simulink model "SF054A_PwrpkCmpbltyChk"  (R2013b)
settings: Solver=FixedStepDiscrete  SolverMode=SingleTasking  StartTime=0.0  StopTime=1  FixedStep=0.1  RelTol=1e-3
values from neighbouring files (symbols this model uses):
  CNVTOCNT_CNTPERMILLISEC_U32 = DataDict.Constant    [SF054A_PwrpkCmpbltyChk_DataDict.m]
  CORRLNFLTBIT2_CNT_U08 = DataDict.Constant    [SF054A_PwrpkCmpbltyChk_DataDict.m]
  CORRLNGEARIDFLTBIT3_CNT_U08 = DataDict.Constant    [SF054A_PwrpkCmpbltyChk_DataDict.m]
  GEARID1INVLBIT0_CNT_U08 = DataDict.Constant    [SF054A_PwrpkCmpbltyChk_DataDict.m]
  GEARID2INVLBIT1_CNT_U08 = DataDict.Constant    [SF054A_PwrpkCmpbltyChk_DataDict.m]
  NODEBSTEP_CNT_U16 = DataDict.Constant    [SF054A_PwrpkCmpbltyChk_DataDict.m]
  NOFAULT_CNT_U08 = DataDict.Constant    [SF054A_PwrpkCmpbltyChk_DataDict.m]
  PwrpkCmpbltyChkGearId = DataDict.Calibration    [SF054A_PwrpkCmpbltyChk_DataDict.m]
  TMRTHD_MILLISEC_U32 = DataDict.Constant    [SF054A_PwrpkCmpbltyChk_DataDict.m]
undefined symbols (not defined in the file or in its folder): NtcNr1, NtcSts1, SigQlfr1
libraries: simulink x10
(part 2 of 3)

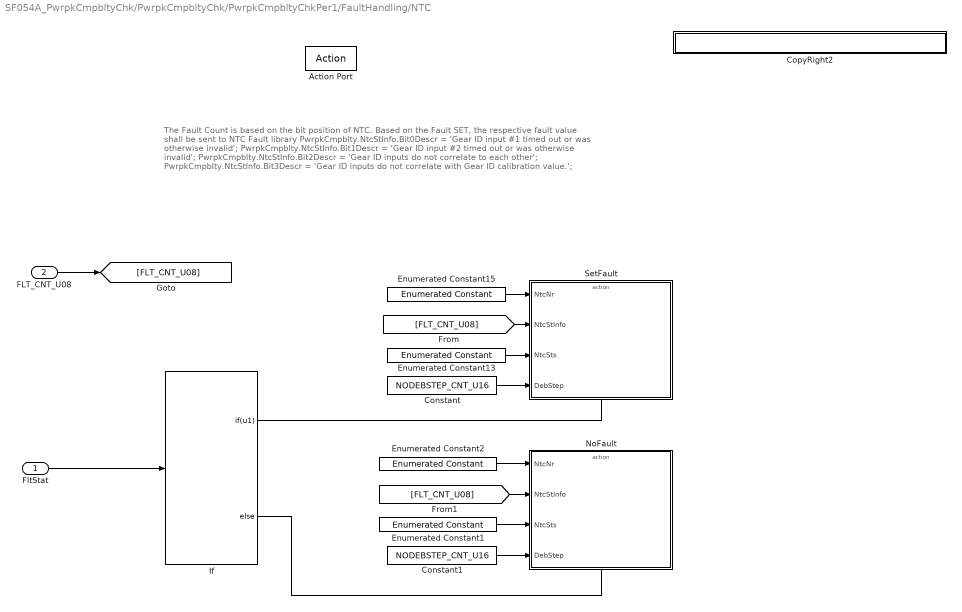
== system SF054A_PwrpkCmpbltyChk/PwrpkCmpbltyChk/PwrpkCmpbltyChkPer1/FaultHandling/NTC ==
  note: The Fault Count is based on the bit position of NTC. Based on the Fault SET, the respective fault value shall be sent to NTC Fault library
      |
      | PwrpkCmpblty.NtcStInfo.Bit0Descr = 'Gear ID input #1 timed out or was otherwise invalid';
      | PwrpkCmpblty.NtcStInfo.Bit1Descr = 'Gear ID input #2 timed out or was otherwise invalid';
      | PwrpkCmpblty.NtcStInfo.Bit2Descr = 'Gear ID inputs do not correlate to each other';
      | PwrpkCmpblty.NtcStInfo.Bit3Descr = 'Gear ID inputs do not correlate with Gear ID calibration value.';
  FltStat : Inport  RequirementInfo="{'linktype_rmi_doors' '0000baba (/E-STEER Core/SubSystem Specifications/Application Functions/SF054A Powerpack Compatibility Check)' '#SF054A_94' 'true' 'REQ:  SF054A_94' '' ; 'linktype_rmi_doors' '0000baba (/E-STEER Core/SubSystem Specifications/Application Functions/SF054A Powerpack Compatibility Check)' '#SF054A_95' 'true' 'REQ:  SF054A_95' '' ; 'linktype_rmi_doors' '0000baba (/E-STEER Core/SubSystem Specifications/Application Functions/SF054A Powerpack Compatibility Check)' '#SF054A_96' 'true' 'REQ:  SF054A_96' '' } %GIDa_d1321426_f376_4e74_abf1_ce402bb86bea"
  FLT_CNT_U08 : Inport  RequirementInfo="{'linktype_rmi_doors' '0000baba (/E-STEER Core/SubSystem Specifications/Application Functions/SF054A Powerpack Compatibility Check)' '#SF054A_94' 'true' 'REQ:  SF054A_94' '' ; 'linktype_rmi_doors' '0000baba (/E-STEER Core/SubSystem Specifications/Application Functions/SF054A Powerpack Compatibility Check)' '#SF054A_95' 'true' 'REQ:  SF054A_95' '' ; 'linktype_rmi_doors' '0000baba (/E-STEER Core/SubSystem Specifications/Application Functions/SF054A Powerpack Compatibility Check)' '#SF054A_96' 'true' 'REQ:  SF054A_96' '' } %GIDa_a4ede8dd_1dc7_48ae_adab_c593f70f9e10"  Port=2
  Action Port : ActionPort  ActionType=then
  Constant : Constant  Value=NODEBSTEP_CNT_U16
  Constant1 : Constant  Value=NODEBSTEP_CNT_U16
  CopyRight2 : Subsystem  Description=|  mask(Copyright Information){none=on}
      | Copyright info block.                                               
      |                                                                     
      | Place copyright information at the top of every subsystem in design.
      mask prompts: none "No parameters"
      mask help: Place copyright information at the top of every subsystem in design.
      mask Display:
      | NxtrConf = 'Nexteer Confidential';
      | 
      | sys = bdroot; %handle for the current model ("system")
      | first = get_param(sys,'Created');
      | if(isempty(first))
      |     first = datestr(now,'yyyy');
      | else
      |     first = first(end-3:end);  %year is last four digits
      | end
      | 
      | last = get_param(sys,'LastModifiedDate');
      | if isempty(last)
      |     last = datestr(now,'yyyy');
      | else
      |     last = last(end-3:end);
      | end
      | 
      | if strcmp(first,last)
      |     fprintf('%s -- Copyright %s Nexteer',NxtrConf,first)
      | else
      |     fprintf('%s -- %s%s- %s Nexteer',NxtrConf,char(169),first,last)
      | end
  Enumerated Constant1 : simulink/Sources/Enumerated Constant  RequirementInfo="{'linktype_rmi_doors' '0000ba59 (/E-STEER Core/SubSystem Specifications/Application Functions/SF011A Learned EOT Limits)' '#SF011A_147' 'true' 'REQ:  SF011A_147' '' ; 'linktype_rmi_doors' '0000baba (/E-STEER Core/SubSystem Specifications/Application Functions/SF054A Powerpack Compatibility Check)' '#SF054A_94' 'true' 'REQ:  SF054A_94' '' ; 'linktype_rmi_doors' '0000baba (/E-STEER Core/SubSystem Specifications/Application Functions/SF054A Powerpack Compatibility Check)' '#SF054A_95' 'true' 'REQ:  SF054A_95' '' ; 'linktype_rmi_doors' '0000baba (/E-STEER Core/SubSystem Specifications/Application Functions/SF054A Powerpack Compatibility Check)' '#SF054A_96' 'true' 'REQ:  SF054A_96' '' ; 'linktype_rmi_doors' '0000baba (/E-STEER Core/SubSystem Specifications/Application Functions/SF054A Powerpack Compatibility Check)' '#SF054A_93' 'true' 'REQ:  SF054A_93' '' ; 'linktype_rmi_doors' '0000baba (/E-STEER Core/SubSystem Specifications/Application Functions/SF054A Powerpack Compatibility Check)' '#SF054A_97' 'true' 'REQ:  SF054A_97' '' } %GIDa_76a10143_d7e5_4556_a877_13f786568e17"  OutDataTypeStr=Enum: NtcSts1  Value=NtcSts1.NTCSTS_PASSD  SampleTime=inf
  Enumerated Constant13 : simulink/Sources/Enumerated Constant  RequirementInfo="{'linktype_rmi_doors' '0000ba59 (/E-STEER Core/SubSystem Specifications/Application Functions/SF011A Learned EOT Limits)' '#SF011A_147' 'true' 'REQ:  SF011A_147' '' ; 'linktype_rmi_doors' '0000baba (/E-STEER Core/SubSystem Specifications/Application Functions/SF054A Powerpack Compatibility Check)' '#SF054A_94' 'true' 'REQ:  SF054A_94' '' ; 'linktype_rmi_doors' '0000baba (/E-STEER Core/SubSystem Specifications/Application Functions/SF054A Powerpack Compatibility Check)' '#SF054A_95' 'true' 'REQ:  SF054A_95' '' ; 'linktype_rmi_doors' '0000baba (/E-STEER Core/SubSystem Specifications/Application Functions/SF054A Powerpack Compatibility Check)' '#SF054A_96' 'true' 'REQ:  SF054A_96' '' } %GIDa_90bc376e_b768_4a6f_b02b_6410e016d981"  OutDataTypeStr=Enum: NtcSts1  Value=NtcSts1.NTCSTS_FAILD  SampleTime=inf
  Enumerated Constant15 : simulink/Sources/Enumerated Constant  RequirementInfo="{'linktype_rmi_doors' '0000ba59 (/E-STEER Core/SubSystem Specifications/Application Functions/SF011A Learned EOT Limits)' '#SF011A_147' 'true' 'REQ:  SF011A_147' '' } %GIDa_98664301_0d49_4c1a_b13b_e4ddba13ec9c"  OutDataTypeStr=Enum: NtcNr1  Value=NtcNr1.NTCNR_0X1F1  SampleTime=inf
  Enumerated Constant2 : simulink/Sources/Enumerated Constant  RequirementInfo="{'linktype_rmi_doors' '0000ba59 (/E-STEER Core/SubSystem Specifications/Application Functions/SF011A Learned EOT Limits)' '#SF011A_147' 'true' 'REQ:  SF011A_147' '' ; 'linktype_rmi_doors' '0000baba (/E-STEER Core/SubSystem Specifications/Application Functions/SF054A Powerpack Compatibility Check)' '#SF054A_94' 'true' 'REQ:  SF054A_94' '' ; 'linktype_rmi_doors' '0000baba (/E-STEER Core/SubSystem Specifications/Application Functions/SF054A Powerpack Compatibility Check)' '#SF054A_95' 'true' 'REQ:  SF054A_95' '' ; 'linktype_rmi_doors' '0000baba (/E-STEER Core/SubSystem Specifications/Application Functions/SF054A Powerpack Compatibility Check)' '#SF054A_96' 'true' 'REQ:  SF054A_96' '' ; 'linktype_rmi_doors' '0000baba (/E-STEER Core/SubSystem Specifications/Application Functions/SF054A Powerpack Compatibility Check)' '#SF054A_93' 'true' 'REQ:  SF054A_93' '' ; 'linktype_rmi_doors' '0000baba (/E-STEER Core/SubSystem Specifications/Application Functions/SF054A Powerpack Compatibility Check)' '#SF054A_97' 'true' 'REQ:  SF054A_97' '' } %GIDa_e47249a4_767f_41c6_83fc_25906c6d5740"  OutDataTypeStr=Enum: NtcNr1  Value=NtcNr1.NTCNR_0X1F1  SampleTime=inf
  If : If  RequirementInfo="{'linktype_rmi_doors' '0000baba (/E-STEER Core/SubSystem Specifications/Application Functions/SF054A Powerpack Compatibility Check)' '#SF054A_93' 'true' 'REQ:  SF054A_93' '' ; 'linktype_rmi_doors' '0000baba (/E-STEER Core/SubSystem Specifications/Application Functions/SF054A Powerpack Compatibility Check)' '#SF054A_97' 'true' 'REQ:  SF054A_97' '' ; 'linktype_rmi_doors' '0000baba (/E-STEER Core/SubSystem Specifications/Application Functions/SF054A Powerpack Compatibility Check)' '#SF054A_94' 'true' 'REQ:  SF054A_94' '' ; 'linktype_rmi_doors' '0000baba (/E-STEER Core/SubSystem Specifications/Application Functions/SF054A Powerpack Compatibility Check)' '#SF054A_95' 'true' 'REQ:  SF054A_95' '' ; 'linktype_rmi_doors' '0000baba (/E-STEER Core/SubSystem Specifications/Application Functions/SF054A Powerpack Compatibility Check)' '#SF054A_96' 'true' 'REQ:  SF054A_96' '' } %GIDa_5ebd1fa8_c02e_40bb_a2aa_3fc1e27259c9"  IfExpression=u1
  NoFault : Subsystem  RequirementInfo="{'linktype_rmi_doors' '0000baba (/E-STEER Core/SubSystem Specifications/Application Functions/SF054A Powerpack Compatibility Check)' '#SF054A_94' 'true' 'REQ:  SF054A_94' '' ; 'linktype_rmi_doors' '0000baba (/E-STEER Core/SubSystem Specifications/Application Functions/SF054A Powerpack Compatibility Check)' '#SF054A_95' 'true' 'REQ:  SF054A_95' '' ; 'linktype_rmi_doors' '0000baba (/E-STEER Core/SubSystem Specifications/Application Functions/SF054A Powerpack Compatibility Check)' '#SF054A_96' 'true' 'REQ:  SF054A_96' '' ; 'linktype_rmi_doors' '0000baba (/E-STEER Core/SubSystem Specifications/Application Functions/SF054A Powerpack Compatibility Check)' '#SF054A_93' 'true' 'REQ:  SF054A_93' '' ; 'linktype_rmi_doors' '0000baba (/E-STEER Core/SubSystem Specifications/Application Functions/SF054A Powerpack Compatibility Check)' '#SF054A_97' 'true' 'REQ:  SF054A_97' '' } %GIDa_9ffc1e70_19a3_4cc1_b8dc_1508988df6dd"  mask(SetNTC){}
      mask help: SetNTC library block
  SetFault : Subsystem  RequirementInfo="{'linktype_rmi_doors' '0000baba (/E-STEER Core/SubSystem Specifications/Application Functions/SF054A Powerpack Compatibility Check)' '#SF054A_93' 'true' 'REQ:  SF054A_93' '' ; 'linktype_rmi_doors' '0000baba (/E-STEER Core/SubSystem Specifications/Application Functions/SF054A Powerpack Compatibility Check)' '#SF054A_97' 'true' 'REQ:  SF054A_97' '' ; 'linktype_rmi_doors' '0000baba (/E-STEER Core/SubSystem Specifications/Application Functions/SF054A Powerpack Compatibility Check)' '#SF054A_94' 'true' 'REQ:  SF054A_94' '' ; 'linktype_rmi_doors' '0000baba (/E-STEER Core/SubSystem Specifications/Application Functions/SF054A Powerpack Compatibility Check)' '#SF054A_95' 'true' 'REQ:  SF054A_95' '' ; 'linktype_rmi_doors' '0000baba (/E-STEER Core/SubSystem Specifications/Application Functions/SF054A Powerpack Compatibility Check)' '#SF054A_96' 'true' 'REQ:  SF054A_96' '' } %GIDa_5c8bf209_0d3d_49fa_8c93_879ef1e5ed4e"  mask(SetNTC){}
      mask help: SetNTC library block
  wires:
  Enumerated Constant15/1 -> SetFault/1(NtcNr)
  Enumerated Constant13/1 -> SetFault/3(NtcSts)
  Constant/1 -> SetFault/4(DebStep)
  [FLT_CNT_U08] -> SetFault/2(NtcStInfo)
  If/1 -> SetFault/Action
  Enumerated Constant2/1 -> NoFault/1(NtcNr)
  Enumerated Constant1/1 -> NoFault/3(NtcSts)
  Constant1/1 -> NoFault/4(DebStep)
  [FLT_CNT_U08] -> NoFault/2(NtcStInfo)
  If/2 -> NoFault/Action
  FltStat/1 -> If/1
  FLT_CNT_U08/1 -> [FLT_CNT_U08]

== system SF054A_PwrpkCmpbltyChk/PwrpkCmpbltyChk/PwrpkCmpbltyChkPer1/FaultHandling/NTCCheck ==
  FltStat : Inport  RequirementInfo="{'linktype_rmi_doors' '0000baba (/E-STEER Core/SubSystem Specifications/Application Functions/SF054A Powerpack Compatibility Check)' '#SF054A_91' 'true' 'REQ:  SF054A_91' '' ; 'linktype_rmi_doors' '0000baba (/E-STEER Core/SubSystem Specifications/Application Functions/SF054A Powerpack Compatibility Check)' '#SF054A_98' 'true' 'REQ:  SF054A_98' '' } %GIDa_cd991dcd_1012_4078_b2f9_adfb3d5191aa"
  Constant : Constant  RequirementInfo="{'linktype_rmi_doors' '0000baba (/E-STEER Core/SubSystem Specifications/Application Functions/SF054A Powerpack Compatibility Check)' '#SF054A_91' 'true' 'REQ:  SF054A_91' '' ; 'linktype_rmi_doors' '0000baba (/E-STEER Core/SubSystem Specifications/Application Functions/SF054A Powerpack Compatibility Check)' '#SF054A_98' 'true' 'REQ:  SF054A_98' '' } %GIDa_b6b6c8fe_27bd_4710_8193_37bbd19d7a9e"
  Enumerated Constant1 : simulink/Sources/Enumerated Constant  RequirementInfo="{'linktype_rmi_doors' '0000baba (/E-STEER Core/SubSystem Specifications/Application Functions/SF054A Powerpack Compatibility Check)' '#SF054A_91' 'true' 'REQ:  SF054A_91' '' ; 'linktype_rmi_doors' '0000baba (/E-STEER Core/SubSystem Specifications/Application Functions/SF054A Powerpack Compatibility Check)' '#SF054A_98' 'true' 'REQ:  SF054A_98' '' } %GIDa_7ed6285f_7121_49e3_927a_e109339fc9b9"  OutDataTypeStr=Enum: SigQlfr1  Value=SigQlfr1.SIGQLFR_PASSD  SampleTime=inf
  Enumerated Constant3 : simulink/Sources/Enumerated Constant  RequirementInfo="{'linktype_rmi_doors' '0000baba (/E-STEER Core/SubSystem Specifications/Application Functions/SF054A Powerpack Compatibility Check)' '#SF054A_91' 'true' 'REQ:  SF054A_91' '' ; 'linktype_rmi_doors' '0000baba (/E-STEER Core/SubSystem Specifications/Application Functions/SF054A Powerpack Compatibility Check)' '#SF054A_98' 'true' 'REQ:  SF054A_98' '' } %GIDa_ae37c846_cbb7_4a30_8716_1da98cb1c54b"  OutDataTypeStr=Enum: NtcNr1  Value=NtcNr1.NTCNR_0X1F1  SampleTime=inf
  Enumerated Constant4 : simulink/Sources/Enumerated Constant  RequirementInfo="{'linktype_rmi_doors' '0000baba (/E-STEER Core/SubSystem Specifications/Application Functions/SF054A Powerpack Compatibility Check)' '#SF054A_91' 'true' 'REQ:  SF054A_91' '' ; 'linktype_rmi_doors' '0000baba (/E-STEER Core/SubSystem Specifications/Application Functions/SF054A Powerpack Compatibility Check)' '#SF054A_98' 'true' 'REQ:  SF054A_98' '' } %GIDa_9ccbda32_b0ec_468a_9ed5_5f897a56dcc4"  OutDataTypeStr=Enum: SigQlfr1  Value=SigQlfr1.SIGQLFR_PASSD  SampleTime=inf
  GetNtcQlfrSts : Subsystem  RequirementInfo="{'linktype_rmi_doors' '0000baba (/E-STEER Core/SubSystem Specifications/Application Functions/SF054A Powerpack Compatibility Check)' '#SF054A_91' 'true' 'REQ:  SF054A_91' '' ; 'linktype_rmi_doors' '0000baba (/E-STEER Core/SubSystem Specifications/Application Functions/SF054A Powerpack Compatibility Check)' '#SF054A_98' 'true' 'REQ:  SF054A_98' '' } %GIDa_63a61b2e_15bc_4085_be85_8a45fba3da91"  Priority=0  TreatAsAtomicUnit=on  mask(GetNTC){}
      mask help: GetNTC library block
      settings: RTWSystemCode=Inline
  If : If  RequirementInfo="{'linktype_rmi_doors' '0000baba (/E-STEER Core/SubSystem Specifications/Application Functions/SF054A Powerpack Compatibility Check)' '#SF054A_91' 'true' 'REQ:  SF054A_91' '' ; 'linktype_rmi_doors' '0000baba (/E-STEER Core/SubSystem Specifications/Application Functions/SF054A Powerpack Compatibility Check)' '#SF054A_98' 'true' 'REQ:  SF054A_98' '' } %GIDa_6f272258_94a1_4eea_8ab6_e33777d6ad2e"  Priority=1  IfExpression=u1  ShowElse=off
  Logical Operator : Logic  RequirementInfo="{'linktype_rmi_doors' '0000baba (/E-STEER Core/SubSystem Specifications/Application Functions/SF054A Powerpack Compatibility Check)' '#SF054A_91' 'true' 'REQ:  SF054A_91' '' ; 'linktype_rmi_doors' '0000baba (/E-STEER Core/SubSystem Specifications/Application Functions/SF054A Powerpack Compatibility Check)' '#SF054A_98' 'true' 'REQ:  SF054A_98' '' } %GIDa_29bb41fa_cbd1_428c_8cf2_147e2dfe02ab"  Operator=OR  AllPortsSameDT=off  OutDataTypeStr=boolean
  Logical Operator1 : Logic  RequirementInfo="{'linktype_rmi_doors' '0000baba (/E-STEER Core/SubSystem Specifications/Application Functions/SF054A Powerpack Compatibility Check)' '#SF054A_91' 'true' 'REQ:  SF054A_91' '' ; 'linktype_rmi_doors' '0000baba (/E-STEER Core/SubSystem Specifications/Application Functions/SF054A Powerpack Compatibility Check)' '#SF054A_98' 'true' 'REQ:  SF054A_98' '' } %GIDa_27601766_4d47_46cd_835d_6e2f4316db1e"  AllPortsSameDT=off  OutDataTypeStr=boolean
  NtcStsChk : RelationalOperator  RequirementInfo="{'linktype_rmi_doors' '0000baba (/E-STEER Core/SubSystem Specifications/Application Functions/SF054A Powerpack Compatibility Check)' '#SF054A_91' 'true' 'REQ:  SF054A_91' '' ; 'linktype_rmi_doors' '0000baba (/E-STEER Core/SubSystem Specifications/Application Functions/SF054A Powerpack Compatibility Check)' '#SF054A_98' 'true' 'REQ:  SF054A_98' '' } %GIDa_b3194a09_2e5a_47be_940a_7a93a9f9800c"  Operator=~=  OutDataTypeStr=boolean
  NtcStsChk1 : RelationalOperator  RequirementInfo="{'linktype_rmi_doors' '0000baba (/E-STEER Core/SubSystem Specifications/Application Functions/SF054A Powerpack Compatibility Check)' '#SF054A_91' 'true' 'REQ:  SF054A_91' '' ; 'linktype_rmi_doors' '0000baba (/E-STEER Core/SubSystem Specifications/Application Functions/SF054A Powerpack Compatibility Check)' '#SF054A_98' 'true' 'REQ:  SF054A_98' '' } %GIDa_82d14e30_4785_436e_ab50_a0d52d13e43f"  Operator===  OutDataTypeStr=boolean
  NtcStsChk2 : RelationalOperator  RequirementInfo="{'linktype_rmi_doors' '0000baba (/E-STEER Core/SubSystem Specifications/Application Functions/SF054A Powerpack Compatibility Check)' '#SF054A_91' 'true' 'REQ:  SF054A_91' '' ; 'linktype_rmi_doors' '0000baba (/E-STEER Core/SubSystem Specifications/Application Functions/SF054A Powerpack Compatibility Check)' '#SF054A_98' 'true' 'REQ:  SF054A_98' '' } %GIDa_f955f7c9_8f8a_47c5_a799_e283ca9a9948"  Operator===  OutDataTypeStr=boolean
  NTC_Condition : Outport  RequirementInfo="{'linktype_rmi_doors' '0000baba (/E-STEER Core/SubSystem Specifications/Application Functions/SF054A Powerpack Compatibility Check)' '#SF054A_91' 'true' 'REQ:  SF054A_91' '' ; 'linktype_rmi_doors' '0000baba (/E-STEER Core/SubSystem Specifications/Application Functions/SF054A Powerpack Compatibility Check)' '#SF054A_98' 'true' 'REQ:  SF054A_98' '' } %GIDa_f2a5627a_783c_4d45_b613_59ba6ee0c185"
  wires:
  Enumerated Constant4/1 -> NtcStsChk/2
  Enumerated Constant3/1 -> GetNtcQlfrSts/1(NtcNr)
  GetNtcQlfrSts/1(NtcQlfr) -> NtcStsChk/1, NtcStsChk1/1
  Enumerated Constant1/1 -> NtcStsChk1/2
  NtcStsChk/1 -> Logical Operator/1
  Logical Operator/1 -> If/1
  If/1 -> NTC_Condition/1
  FltStat/1 -> NtcStsChk2/2
  Constant/1 -> NtcStsChk2/1
  NtcStsChk1/1 -> Logical Operator1/1
  NtcStsChk2/1 -> Logical Operator1/2
  Logical Operator1/1 -> Logical Operator/2

== system SF054A_PwrpkCmpbltyChk/PwrpkCmpbltyChk/PwrpkCmpbltyChkPer1/FaultDetection/CorrlnChk/CopyRight2 ==

== system SF054A_PwrpkCmpbltyChk/PwrpkCmpbltyChk/PwrpkCmpbltyChkPer1/FaultDetection/CorrlnChk/CorrlnFltChk ==
  GearIdn1 : Inport
  GearIdn2 : Inport  Port=2
  Action Port : ActionPort  ActionType=then
  CopyRight2 : Subsystem  Description=|  mask(Copyright Information){none=on}
      | Copyright info block.                                               
      |                                                                     
      | Place copyright information at the top of every subsystem in design.
      mask prompts: none "No parameters"
      mask help: Place copyright information at the top of every subsystem in design.
      mask Display:
      | NxtrConf = 'Nexteer Confidential';
      | 
      | sys = bdroot; %handle for the current model ("system")
      | first = get_param(sys,'Created');
      | if(isempty(first))
      |     first = datestr(now,'yyyy');
      | else
      |     first = first(end-3:end);  %year is last four digits
      | end
      | 
      | last = get_param(sys,'LastModifiedDate');
      | if isempty(last)
      |     last = datestr(now,'yyyy');
      | else
      |     last = last(end-3:end);
      | end
      | 
      | if strcmp(first,last)
      |     fprintf('%s -- Copyright %s Nexteer',NxtrConf,first)
      | else
      |     fprintf('%s -- %s%s- %s Nexteer',NxtrConf,char(169),first,last)
      | end
  GearIdCorrlnChk : Subsystem  RequirementInfo="{'linktype_rmi_doors' '0000baba (/E-STEER Core/SubSystem Specifications/Application Functions/SF054A Powerpack Compatibility Check)' '#SF054A_69' 'true' 'REQ:  SF054A_69' '' } %GIDa_fbed16ac_51b0_425e_93d9_51fb01c78695"  TreatAsAtomicUnit=on
  SigCorrlnChk : Subsystem  RequirementInfo="{'linktype_rmi_doors' '0000baba (/E-STEER Core/SubSystem Specifications/Application Functions/SF054A Powerpack Compatibility Check)' '#SF054A_67' 'true' 'REQ:  SF054A_67' '' } %GIDa_4edc7e58_d267_41ea_8f9b_2f7686a22c38"  TreatAsAtomicUnit=on
  GearIdCorrlnFltStat : Outport
  CorrlnFltStat : Outport  Port=2
  CorrlnFltCnt : Outport  Port=3
  GearIdCorrlnFltCnt : Outport  Port=4
  wires:
  GearIdn2/1 -> GearIdCorrlnChk/1(GearIdn2), SigCorrlnChk/2(GearIdn2)
  GearIdn1/1 -> GearIdCorrlnChk/2(GearIdn1), SigCorrlnChk/1(GearIdn1)
  GearIdCorrlnChk/1(GearIdCorrlnFltStat) -> GearIdCorrlnFltStat/1
  SigCorrlnChk/1(CorrlnFltStat) -> CorrlnFltStat/1
  SigCorrlnChk/2(CorrlnFltCnt) -> CorrlnFltCnt/1
  GearIdCorrlnChk/2(GearIdCorrlnFltCnt) -> GearIdCorrlnFltCnt/1

== system SF054A_PwrpkCmpbltyChk/PwrpkCmpbltyChk/PwrpkCmpbltyChkPer1/FaultDetection/CorrlnChk/Default ==
  Action Port : ActionPort  ActionType=else
  Constant : Constant  Value=false  OutDataTypeStr=boolean
  Constant1 : Constant  Value=false  OutDataTypeStr=boolean
  Constant2 : Constant  Value=0  OutDataTypeStr=uint8
  Constant3 : Constant  Value=0  OutDataTypeStr=uint8
  CopyRight2 : Subsystem  Description=|  mask(Copyright Information){none=on}
      | Copyright info block.                                               
      |                                                                     
      | Place copyright information at the top of every subsystem in design.
      mask prompts: none "No parameters"
      mask help: Place copyright information at the top of every subsystem in design.
      mask Display:
      | NxtrConf = 'Nexteer Confidential';
      | 
      | sys = bdroot; %handle for the current model ("system")
      | first = get_param(sys,'Created');
      | if(isempty(first))
      |     first = datestr(now,'yyyy');
      | else
      |     first = first(end-3:end);  %year is last four digits
      | end
      | 
      | last = get_param(sys,'LastModifiedDate');
      | if isempty(last)
      |     last = datestr(now,'yyyy');
      | else
      |     last = last(end-3:end);
      | end
      | 
      | if strcmp(first,last)
      |     fprintf('%s -- Copyright %s Nexteer',NxtrConf,first)
      | else
      |     fprintf('%s -- %s%s- %s Nexteer',NxtrConf,char(169),first,last)
      | end
  GearIdCorrlnFltCnt : Outport
  CorrlnFltCnt : Outport  Port=2
  CorrlnFltStat : Outport  Port=3
  GearIdCorrlnFltStat : Outport  Port=4
  wires:
  Constant/1 -> CorrlnFltStat/1
  Constant1/1 -> GearIdCorrlnFltStat/1
  Constant2/1 -> CorrlnFltCnt/1
  Constant3/1 -> GearIdCorrlnFltCnt/1

== system SF054A_PwrpkCmpbltyChk/PwrpkCmpbltyChk/PwrpkCmpbltyChkPer1/FaultDetection/GearSigChk/CopyRight2 ==

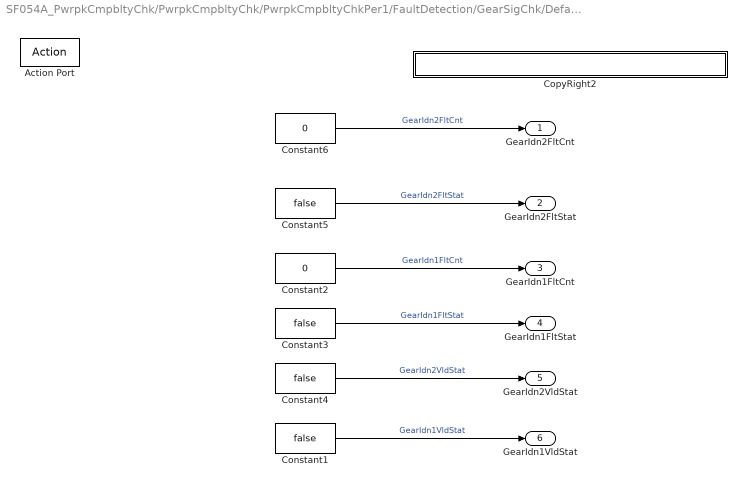
== system SF054A_PwrpkCmpbltyChk/PwrpkCmpbltyChk/PwrpkCmpbltyChkPer1/FaultDetection/GearSigChk/Default ==
  Action Port : ActionPort  ActionType=else
  Constant{1,3..5} (4 alike) : Constant  Value=false  OutDataTypeStr=boolean
      settings: AttributesFormatString=%<OutDataTypeStr>
  Constant2 : Constant  Value=0  OutDataTypeStr=uint8
      settings: AttributesFormatString=%<OutDataTypeStr>
  Constant6 : Constant  Value=0  OutDataTypeStr=uint8
      settings: AttributesFormatString=%<OutDataTypeStr>
  CopyRight2 : Subsystem  Description=|  mask(Copyright Information){none=on}
      | Copyright info block.                                               
      |                                                                     
      | Place copyright information at the top of every subsystem in design.
      mask prompts: none "No parameters"
      mask help: Place copyright information at the top of every subsystem in design.
      mask Display:
      | NxtrConf = 'Nexteer Confidential';
      | 
      | sys = bdroot; %handle for the current model ("system")
      | first = get_param(sys,'Created');
      | if(isempty(first))
      |     first = datestr(now,'yyyy');
      | else
      |     first = first(end-3:end);  %year is last four digits
      | end
      | 
      | last = get_param(sys,'LastModifiedDate');
      | if isempty(last)
      |     last = datestr(now,'yyyy');
      | else
      |     last = last(end-3:end);
      | end
      | 
      | if strcmp(first,last)
      |     fprintf('%s -- Copyright %s Nexteer',NxtrConf,first)
      | else
      |     fprintf('%s -- %s%s- %s Nexteer',NxtrConf,char(169),first,last)
      | end
  GearIdn2FltCnt : Outport
  GearIdn2FltStat : Outport  Port=2
  GearIdn1FltCnt : Outport  Port=3
  GearIdn1FltStat : Outport  Port=4
  GearIdn2VldStat : Outport  Port=5
  GearIdn1VldStat : Outport  Port=6
  wires:
  Constant1/1 -> GearIdn1VldStat/1  "GearIdn1VldStat"
  Constant3/1 -> GearIdn1FltStat/1  "GearIdn1FltStat"
  Constant2/1 -> GearIdn1FltCnt/1  "GearIdn1FltCnt"
  Constant4/1 -> GearIdn2VldStat/1  "GearIdn2VldStat"
  Constant5/1 -> GearIdn2FltStat/1  "GearIdn2FltStat"
  Constant6/1 -> GearIdn2FltCnt/1  "GearIdn2FltCnt"

== system SF054A_PwrpkCmpbltyChk/PwrpkCmpbltyChk/PwrpkCmpbltyChkPer1/FaultDetection/GearSigChk/GearSigVldChk ==
  GearIdn1Vld : Inport
  GearIdn2Vld : Inport  Port=2
  Action Port : ActionPort  ActionType=then
  CopyRight2 : Subsystem  Description=|  mask(Copyright Information){none=on}
      | Copyright info block.                                               
      |                                                                     
      | Place copyright information at the top of every subsystem in design.
      mask prompts: none "No parameters"
      mask help: Place copyright information at the top of every subsystem in design.
      mask Display:
      | NxtrConf = 'Nexteer Confidential';
      | 
      | sys = bdroot; %handle for the current model ("system")
      | first = get_param(sys,'Created');
      | if(isempty(first))
      |     first = datestr(now,'yyyy');
      | else
      |     first = first(end-3:end);  %year is last four digits
      | end
      | 
      | last = get_param(sys,'LastModifiedDate');
      | if isempty(last)
      |     last = datestr(now,'yyyy');
      | else
      |     last = last(end-3:end);
      | end
      | 
      | if strcmp(first,last)
      |     fprintf('%s -- Copyright %s Nexteer',NxtrConf,first)
      | else
      |     fprintf('%s -- %s%s- %s Nexteer',NxtrConf,char(169),first,last)
      | end
  GearIdn1 : Subsystem  RequirementInfo="{'linktype_rmi_doors' '0000baba (/E-STEER Core/SubSystem Specifications/Application Functions/SF054A Powerpack Compatibility Check)' '#SF054A_80' 'true' 'REQ:  SF054A_80' '' } %GIDa_9c5e6da7_6f82_4606_90df_0929d56a431b"  TreatAsAtomicUnit=on
  GearIdn2 : Subsystem  RequirementInfo="{'linktype_rmi_doors' '0000baba (/E-STEER Core/SubSystem Specifications/Application Functions/SF054A Powerpack Compatibility Check)' '#SF054A_80' 'true' 'REQ:  SF054A_80' '' } %GIDa_238ccb51_49de_437c_8762_d37e902bfe47"  TreatAsAtomicUnit=on
  GearIdn1VldStat : Outport
  GearIdn2VldStat : Outport  Port=2
  GearIdn1FltStat : Outport  Port=3
  GearIdn1FltCnt : Outport  Port=4
  GearIdn2FltStat : Outport  Port=5
  GearIdn2FltCnt : Outport  Port=6
  wires:
  GearIdn1Vld/1 -> GearIdn1/1(GearIdn1Vld)
  GearIdn2Vld/1 -> GearIdn2/1(GearIdn2Vld)
  GearIdn1/1(GearIdn1FltCnt) -> GearIdn1FltCnt/1  "GearIdn1FltCnt"
  GearIdn1/2(GearIdn1FltStat) -> GearIdn1FltStat/1  "GearIdn1FltStat"
  GearIdn1/3(GearIdn1VldStat) -> GearIdn1VldStat/1  "GearIdn1VldStat"
  GearIdn2/1(GearIdn2FltStat) -> GearIdn2FltStat/1  "GearIdn2FltStat"
  GearIdn2/2(GearIdn2VldStat) -> GearIdn2VldStat/1  "GearIdn2VldStat"
  GearIdn2/3(GearIdn2FltCnt) -> GearIdn2FltCnt/1  "GearIdn2FltCnt"

== system SF054A_PwrpkCmpbltyChk/PwrpkCmpbltyChk/PwrpkCmpbltyChkPer1/FaultDetection/GearSigChk/TmrElpdDetn ==
  GearIdnRefTmr : Inport
  Constant : Constant  Value=TMRTHD_MILLISEC_U32
  Constant1 : Constant  Value=CNVTOCNT_CNTPERMILLISEC_U32
  CopyRight2 : Subsystem  Description=|  mask(Copyright Information){none=on}
      | Copyright info block.                                               
      |                                                                     
      | Place copyright information at the top of every subsystem in design.
      mask prompts: none "No parameters"
      mask help: Place copyright information at the top of every subsystem in design.
      mask Display:
      | NxtrConf = 'Nexteer Confidential';
      | 
      | sys = bdroot; %handle for the current model ("system")
      | first = get_param(sys,'Created');
      | if(isempty(first))
      |     first = datestr(now,'yyyy');
      | else
      |     first = first(end-3:end);  %year is last four digits
      | end
      | 
      | last = get_param(sys,'LastModifiedDate');
      | if isempty(last)
      |     last = datestr(now,'yyyy');
      | else
      |     last = last(end-3:end);
      | end
      | 
      | if strcmp(first,last)
      |     fprintf('%s -- Copyright %s Nexteer',NxtrConf,first)
      | else
      |     fprintf('%s -- %s%s- %s Nexteer',NxtrConf,char(169),first,last)
      | end
  GetTiSpan100MicroSec32bit : Subsystem
  Product : Product
  Relational Operator : RelationalOperator  OutDataTypeStr=boolean
  TimeOut : Outport
  wires:
  GearIdnRefTmr/1 -> GetTiSpan100MicroSec32bit/1(RefTmr)
  GetTiSpan100MicroSec32bit/1(TiSpan) -> Relational Operator/1
  Product/1 -> Relational Operator/2
  Constant/1 -> Product/1
  Constant1/1 -> Product/2
  Relational Operator/1 -> TimeOut/1

== system SF054A_PwrpkCmpbltyChk/PwrpkCmpbltyChk/PwrpkCmpbltyChkPer1/FaultHandling/FaultSelection/CopyRight2 ==

== system SF054A_PwrpkCmpbltyChk/PwrpkCmpbltyChk/PwrpkCmpbltyChkPer1/FaultHandling/NTC/CopyRight2 ==

== system SF054A_PwrpkCmpbltyChk/PwrpkCmpbltyChk/PwrpkCmpbltyChkPer1/FaultHandling/NTC/NoFault ==
  NtcNr : Inport
  NtcStInfo : Inport  Port=2
  NtcSts : Inport  Port=3
  DebStep : Inport  Port=4
  CallDiagMgr : ActionPort  ActionType=else
  SetNtcSts : Subsystem  RequirementInfo={} %GIDa_fda9d135_5219_4b4d_8e9f_98dbb4a93628  TreatAsAtomicUnit=on
      settings: RTWSystemCode=Inline
  wires:
  NtcStInfo/1 -> SetNtcSts/2(NtcStInfo)
  DebStep/1 -> SetNtcSts/4(DebStep)
  NtcSts/1 -> SetNtcSts/3(NtcSts)
  NtcNr/1 -> SetNtcSts/1(NtcNr)  "NtcNr"

== system SF054A_PwrpkCmpbltyChk/PwrpkCmpbltyChk/PwrpkCmpbltyChkPer1/FaultHandling/NTC/SetFault ==
  NtcNr : Inport
  NtcStInfo : Inport  Port=2
  NtcSts : Inport  Port=3
  DebStep : Inport  Port=4
  CallDiagMgr : ActionPort  ActionType=then
  SetNtcSts : Subsystem  RequirementInfo={} %GIDa_fb4c5a2b_2292_42fe_b71f_2e84b053594d  TreatAsAtomicUnit=on
      settings: RTWSystemCode=Inline
  wires:
  NtcNr/1 -> SetNtcSts/1(NtcNr)  "NtcNr"
  NtcSts/1 -> SetNtcSts/3(NtcSts)
  DebStep/1 -> SetNtcSts/4(DebStep)
  NtcStInfo/1 -> SetNtcSts/2(NtcStInfo)

== system SF054A_PwrpkCmpbltyChk/PwrpkCmpbltyChk/PwrpkCmpbltyChkPer1/FaultHandling/NTCCheck/GetNtcQlfrSts ==
  NtcNr : Inport
  CopyRight2 : Subsystem  Description=|  mask(Copyright Information){none=on}
      | Copyright info block.                                               
      |                                                                     
      | Place copyright information at the top of every subsystem in design.
      mask prompts: none "No parameters"
      mask help: Place copyright information at the top of every subsystem in design.
      mask Display:
      | NxtrConf = 'Nexteer Confidential';
      | 
      | sys = bdroot; %handle for the current model ("system")
      | first = get_param(sys,'Created');
      | if(isempty(first))
      |     first = datestr(now,'yyyy');
      | else
      |     first = first(end-3:end);  %year is last four digits
      | end
      | 
      | last = get_param(sys,'LastModifiedDate');
      | if isempty(last)
      |     last = datestr(now,'yyyy');
      | else
      |     last = last(end-3:end);
      | end
      | 
      | if strcmp(first,last)
      |     fprintf('%s -- Copyright %s Nexteer',NxtrConf,first)
      | else
      |     fprintf('%s -- %s%s- %s Nexteer',NxtrConf,char(169),first,last)
      | end
  Data Store Read : DataStoreRead  DataStoreName=NtcQlfr
  Terminator : Terminator
  NtcQlfr : Outport
  wires:
  NtcNr/1 -> Terminator/1
  Data Store Read/1 -> NtcQlfr/1

== system SF054A_PwrpkCmpbltyChk/PwrpkCmpbltyChk/PwrpkCmpbltyChkPer1/FaultDetection/CorrlnChk/CorrlnFltChk/CopyRight2 ==

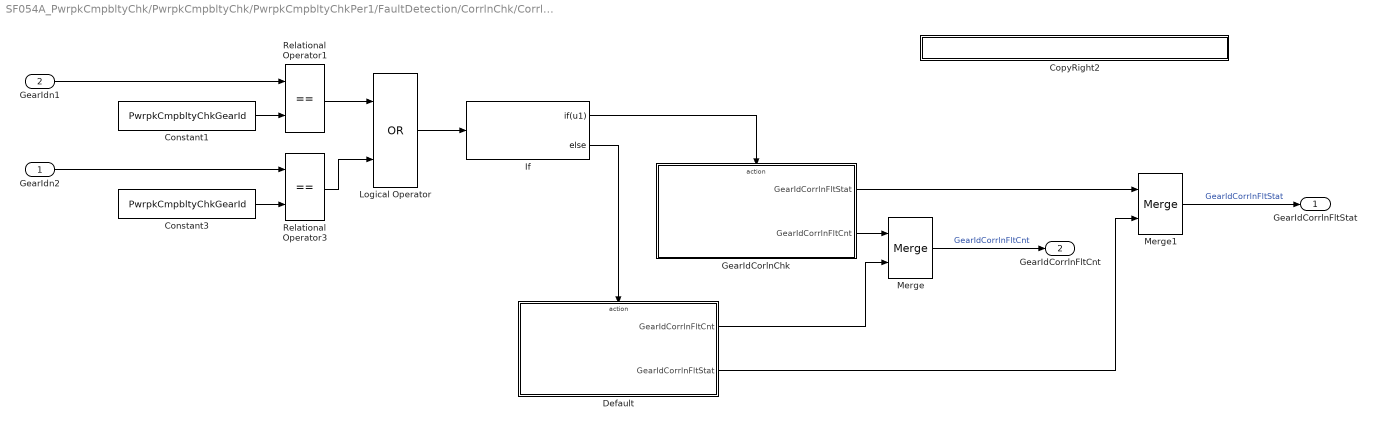
== system SF054A_PwrpkCmpbltyChk/PwrpkCmpbltyChk/PwrpkCmpbltyChkPer1/FaultDetection/CorrlnChk/CorrlnFltChk/GearIdCorrlnChk ==
  GearIdn2 : Inport
  GearIdn1 : Inport  Port=2
  Constant1 : Constant  RequirementInfo="{'linktype_rmi_doors' '0000baba (/E-STEER Core/SubSystem Specifications/Application Functions/SF054A Powerpack Compatibility Check)' '#SF054A_63' 'true' 'REQ:  SF054A_63' '' } %GIDa_3733734c_7d8c_4e6d_be2d_b236cf4ffd0b"  Value=PwrpkCmpbltyChkGearId
  Constant3 : Constant  RequirementInfo="{'linktype_rmi_doors' '0000baba (/E-STEER Core/SubSystem Specifications/Application Functions/SF054A Powerpack Compatibility Check)' '#SF054A_63' 'true' 'REQ:  SF054A_63' '' } %GIDa_d0181d14_c417_4985_90f1_10a4f8105721"  Value=PwrpkCmpbltyChkGearId
  CopyRight2 : Subsystem  Description=|  mask(Copyright Information){none=on}
      | Copyright info block.                                               
      |                                                                     
      | Place copyright information at the top of every subsystem in design.
      mask prompts: none "No parameters"
      mask help: Place copyright information at the top of every subsystem in design.
      mask Display:
      | NxtrConf = 'Nexteer Confidential';
      | 
      | sys = bdroot; %handle for the current model ("system")
      | first = get_param(sys,'Created');
      | if(isempty(first))
      |     first = datestr(now,'yyyy');
      | else
      |     first = first(end-3:end);  %year is last four digits
      | end
      | 
      | last = get_param(sys,'LastModifiedDate');
      | if isempty(last)
      |     last = datestr(now,'yyyy');
      | else
      |     last = last(end-3:end);
      | end
      | 
      | if strcmp(first,last)
      |     fprintf('%s -- Copyright %s Nexteer',NxtrConf,first)
      | else
      |     fprintf('%s -- %s%s- %s Nexteer',NxtrConf,char(169),first,last)
      | end
  Default : Subsystem  TreatAsAtomicUnit=on
  GearIdCorlnChk : Subsystem  TreatAsAtomicUnit=on
  If : If  IfExpression=u1
  Logical Operator : Logic  Operator=OR  AllPortsSameDT=off  OutDataTypeStr=boolean
  Merge : Merge
  Merge1 : Merge
  Relational Operator1 : RelationalOperator  Operator===  OutDataTypeStr=boolean
  Relational Operator3 : RelationalOperator  Operator===  OutDataTypeStr=boolean
  GearIdCorrlnFltStat : Outport
  GearIdCorrlnFltCnt : Outport  Port=2
  wires:
  Relational Operator1/1 -> Logical Operator/1
  Constant3/1 -> Relational Operator3/2
  GearIdn1/1 -> Relational Operator1/1
  Logical Operator/1 -> If/1
  If/1 -> GearIdCorlnChk/Action
  If/2 -> Default/Action
  Default/1(GearIdCorrlnFltCnt) -> Merge/2
  GearIdCorlnChk/2(GearIdCorrlnFltCnt) -> Merge/1
  Merge/1 -> GearIdCorrlnFltCnt/1  "GearIdCorrlnFltCnt"
  GearIdCorlnChk/1(GearIdCorrlnFltStat) -> Merge1/1
  Default/2(GearIdCorrlnFltStat) -> Merge1/2
  Merge1/1 -> GearIdCorrlnFltStat/1  "GearIdCorrlnFltStat"
  Constant1/1 -> Relational Operator1/2
  Relational Operator3/1 -> Logical Operator/2
  GearIdn2/1 -> Relational Operator3/1

== system SF054A_PwrpkCmpbltyChk/PwrpkCmpbltyChk/PwrpkCmpbltyChkPer1/FaultDetection/CorrlnChk/CorrlnFltChk/SigCorrlnChk ==
  GearIdn1 : Inport
  GearIdn2 : Inport  Port=2
  CopyRight2 : Subsystem  Description=|  mask(Copyright Information){none=on}
      | Copyright info block.                                               
      |                                                                     
      | Place copyright information at the top of every subsystem in design.
      mask prompts: none "No parameters"
      mask help: Place copyright information at the top of every subsystem in design.
      mask Display:
      | NxtrConf = 'Nexteer Confidential';
      | 
      | sys = bdroot; %handle for the current model ("system")
      | first = get_param(sys,'Created');
      | if(isempty(first))
      |     first = datestr(now,'yyyy');
      | else
      |     first = first(end-3:end);  %year is last four digits
      | end
      | 
      | last = get_param(sys,'LastModifiedDate');
      | if isempty(last)
      |     last = datestr(now,'yyyy');
      | else
      |     last = last(end-3:end);
      | end
      | 
      | if strcmp(first,last)
      |     fprintf('%s -- Copyright %s Nexteer',NxtrConf,first)
      | else
      |     fprintf('%s -- %s%s- %s Nexteer',NxtrConf,char(169),first,last)
      | end
  CorrelationCheck : Subsystem  TreatAsAtomicUnit=on
  Default : Subsystem  TreatAsAtomicUnit=on
  If : If  IfExpression=u1
  Merge : Merge
  Merge1 : Merge
  Relational Operator : RelationalOperator  Operator===  OutDataTypeStr=boolean
  CorrlnFltStat : Outport
  CorrlnFltCnt : Outport  Port=2
  wires:
  GearIdn1/1 -> Relational Operator/1
  GearIdn2/1 -> Relational Operator/2
  Relational Operator/1 -> If/1
  If/1 -> CorrelationCheck/Action
  If/2 -> Default/Action
  CorrelationCheck/1(CorrlnFltStat) -> Merge/1
  Merge/1 -> CorrlnFltStat/1  "CorrlnFltStat"
  Default/1(CorrlnFltCnt) -> Merge1/2
  CorrelationCheck/2(CorrlnFltCnt) -> Merge1/1
  Default/2(CorrlnFltStat) -> Merge/2
  Merge1/1 -> CorrlnFltCnt/1  "CorrlnFltCnt"

== system SF054A_PwrpkCmpbltyChk/PwrpkCmpbltyChk/PwrpkCmpbltyChkPer1/FaultDetection/CorrlnChk/Default/CopyRight2 ==

== system SF054A_PwrpkCmpbltyChk/PwrpkCmpbltyChk/PwrpkCmpbltyChkPer1/FaultDetection/GearSigChk/Default/CopyRight2 ==

== system SF054A_PwrpkCmpbltyChk/PwrpkCmpbltyChk/PwrpkCmpbltyChkPer1/FaultDetection/GearSigChk/GearSigVldChk/CopyRight2 ==

== system SF054A_PwrpkCmpbltyChk/PwrpkCmpbltyChk/PwrpkCmpbltyChkPer1/FaultDetection/GearSigChk/GearSigVldChk/GearIdn1 ==
  GearIdn1Vld : Inport
  CopyRight2 : Subsystem  Description=|  mask(Copyright Information){none=on}
      | Copyright info block.                                               
      |                                                                     
      | Place copyright information at the top of every subsystem in design.
      mask prompts: none "No parameters"
      mask help: Place copyright information at the top of every subsystem in design.
      mask Display:
      | NxtrConf = 'Nexteer Confidential';
      | 
      | sys = bdroot; %handle for the current model ("system")
      | first = get_param(sys,'Created');
      | if(isempty(first))
      |     first = datestr(now,'yyyy');
      | else
      |     first = first(end-3:end);  %year is last four digits
      | end
      | 
      | last = get_param(sys,'LastModifiedDate');
      | if isempty(last)
      |     last = datestr(now,'yyyy');
      | else
      |     last = last(end-3:end);
      | end
      | 
      | if strcmp(first,last)
      |     fprintf('%s -- Copyright %s Nexteer',NxtrConf,first)
      | else
      |     fprintf('%s -- %s%s- %s Nexteer',NxtrConf,char(169),first,last)
      | end
  Default : Subsystem  TreatAsAtomicUnit=on
  GearId1Vld : Subsystem  TreatAsAtomicUnit=on
  If : If  IfExpression=u1
  Merge : Merge
  Merge1 : Merge
  Merge2 : Merge
  GearIdn1FltCnt : Outport
  GearIdn1FltStat : Outport  Port=2
  GearIdn1VldStat : Outport  Port=3
  wires:
  If/2 -> Default/Action
  GearIdn1Vld/1 -> If/1
  If/1 -> GearId1Vld/Action
  Merge/1 -> GearIdn1FltCnt/1  "GearIdn1FltCnt"
  Default/1(GearIdn1FltCnt) -> Merge/2
  GearId1Vld/3(GearIdn1FltCnt) -> Merge/1
  Default/2(GearIdn1FltStat) -> Merge1/2
  GearId1Vld/2(GearIdn1FltStat) -> Merge1/1
  Merge1/1 -> GearIdn1FltStat/1  "GearIdn1FltStat"
  GearId1Vld/1(GearIdn1VldStat) -> Merge2/1
  Default/3(GearIdn1VldStat) -> Merge2/2
  Merge2/1 -> GearIdn1VldStat/1  "GearIdn1VldStat"

== system SF054A_PwrpkCmpbltyChk/PwrpkCmpbltyChk/PwrpkCmpbltyChkPer1/FaultDetection/GearSigChk/GearSigVldChk/GearIdn2 ==
  GearIdn2Vld : Inport
  CopyRight2 : Subsystem  Description=|  mask(Copyright Information){none=on}
      | Copyright info block.                                               
      |                                                                     
      | Place copyright information at the top of every subsystem in design.
      mask prompts: none "No parameters"
      mask help: Place copyright information at the top of every subsystem in design.
      mask Display:
      | NxtrConf = 'Nexteer Confidential';
      | 
      | sys = bdroot; %handle for the current model ("system")
      | first = get_param(sys,'Created');
      | if(isempty(first))
      |     first = datestr(now,'yyyy');
      | else
      |     first = first(end-3:end);  %year is last four digits
      | end
      | 
      | last = get_param(sys,'LastModifiedDate');
      | if isempty(last)
      |     last = datestr(now,'yyyy');
      | else
      |     last = last(end-3:end);
      | end
      | 
      | if strcmp(first,last)
      |     fprintf('%s -- Copyright %s Nexteer',NxtrConf,first)
      | else
      |     fprintf('%s -- %s%s- %s Nexteer',NxtrConf,char(169),first,last)
      | end
  Default : Subsystem  TreatAsAtomicUnit=on
  GearId1Vld : Subsystem  TreatAsAtomicUnit=on
  If : If  IfExpression=u1
  Merge : Merge
  Merge1 : Merge
  Merge2 : Merge
  GearIdn2FltStat : Outport
  GearIdn2VldStat : Outport  Port=2
  GearIdn2FltCnt : Outport  Port=3
  wires:
  If/1 -> GearId1Vld/Action
  GearIdn2Vld/1 -> If/1
  If/2 -> Default/Action
  GearId1Vld/3(GearIdn2FltCnt) -> Merge/1
  Default/1(GearIdn2FltCnt) -> Merge/2
  Merge/1 -> GearIdn2FltCnt/1  "GearIdn2FltCnt"
  GearId1Vld/2(GearIdn2FltStat) -> Merge1/1
  Default/2(GearIdn2FltStat) -> Merge1/2
  GearId1Vld/1(GearIdn2VldStat) -> Merge2/1
  Default/3(GearIdn2VldStat) -> Merge2/2
  Merge1/1 -> GearIdn2FltStat/1  "GearIdn2FltStat"
  Merge2/1 -> GearIdn2VldStat/1  "GearIdn2VldStat"

== system SF054A_PwrpkCmpbltyChk/PwrpkCmpbltyChk/PwrpkCmpbltyChkPer1/FaultDetection/GearSigChk/TmrElpdDetn/CopyRight2 ==

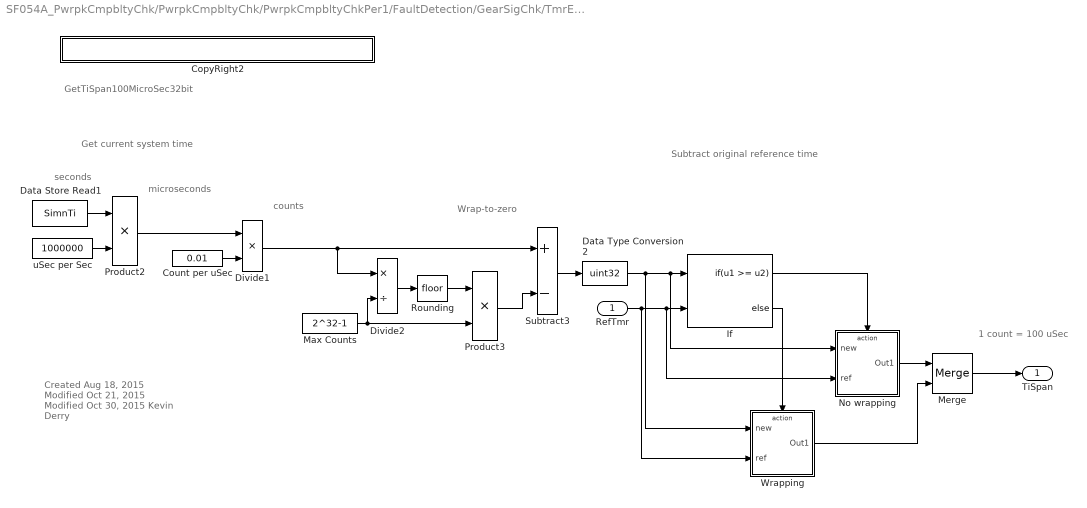
== system SF054A_PwrpkCmpbltyChk/PwrpkCmpbltyChk/PwrpkCmpbltyChkPer1/FaultDetection/GearSigChk/TmrElpdDetn/GetTiSpan100MicroSec32bit ==
  note: Subtract original reference time
  note: seconds
  note: microseconds
  note: counts
  note: Wrap-to-zero
  note: 1 count = 100 uSec
  note: Get current system time
  note: GetTiSpan100MicroSec32bit
  note: Created Aug 18, 2015
      | Modified Oct 21, 2015
      | Modified Oct 30, 2015
      | Kevin Derry
  RefTmr : Inport
  CopyRight2 : Subsystem  Description=|  mask(Copyright Information){none=on}
      | Copyright info block.                                               
      |                                                                     
      | Place copyright information at the top of every subsystem in design.
      mask prompts: none "No parameters"
      mask help: Place copyright information at the top of every subsystem in design.
      mask Display:
      | NxtrConf = 'Nexteer Confidential';
      | 
      | sys = bdroot; %handle for the current model ("system")
      | first = get_param(sys,'Created');
      | if(isempty(first))
      |     first = datestr(now,'yyyy');
      | else
      |     first = first(end-3:end);  %year is last four digits
      | end
      | 
      | last = get_param(sys,'LastModifiedDate');
      | if isempty(last)
      |     last = datestr(now,'yyyy');
      | else
      |     last = last(end-3:end);
      | end
      | 
      | if strcmp(first,last)
      |     fprintf('%s -- Copyright %s Nexteer',NxtrConf,first)
      | else
      |     fprintf('%s -- %s%s- %s Nexteer',NxtrConf,char(169),first,last)
      | end
  Count per uSec : Constant  Value=0.01
  Data Store Read1 : DataStoreRead  DataStoreName=SimnTi
  Data Type Conversion2 : DataTypeConversion  OutDataTypeStr=uint32
  Divide1 : Product  Inputs=**
  Divide2 : Product  Inputs=*/
  If : If  NumInputs=2  IfExpression=u1 >= u2
  Max Counts : Constant  Value=2^32-1
  Merge : Merge
  No wrapping : Subsystem  TreatAsAtomicUnit=on
  Product2 : Product
  Product3 : Product
  Rounding : Rounding
  Subtract3 : Sum  Inputs=+-
  Wrapping : Subsystem  TreatAsAtomicUnit=on
  uSec per Sec : Constant  Value=1000000
  TiSpan : Outport
  wires:
  Wrapping/1(Out1) -> Merge/2
  No wrapping/1(Out1) -> Merge/1
  If/2 -> Wrapping/Action
  If/1 -> No wrapping/Action
  Product3/1 -> Subtract3/2
  Subtract3/1 -> Data Type Conversion2/1
  Rounding/1 -> Product3/1
  Divide2/1 -> Rounding/1
  Max Counts/1 -> Divide2/2, Product3/2
  Divide1/1 -> Divide2/1, Subtract3/1
  Product2/1 -> Divide1/1
  Data Store Read1/1 -> Product2/1
  Count per uSec/1 -> Divide1/2
  uSec per Sec/1 -> Product2/2
  Merge/1 -> TiSpan/1
  RefTmr/1 -> If/2, No wrapping/2(ref), Wrapping/2(ref)
  Data Type Conversion2/1 -> If/1, No wrapping/1(new), Wrapping/1(new)

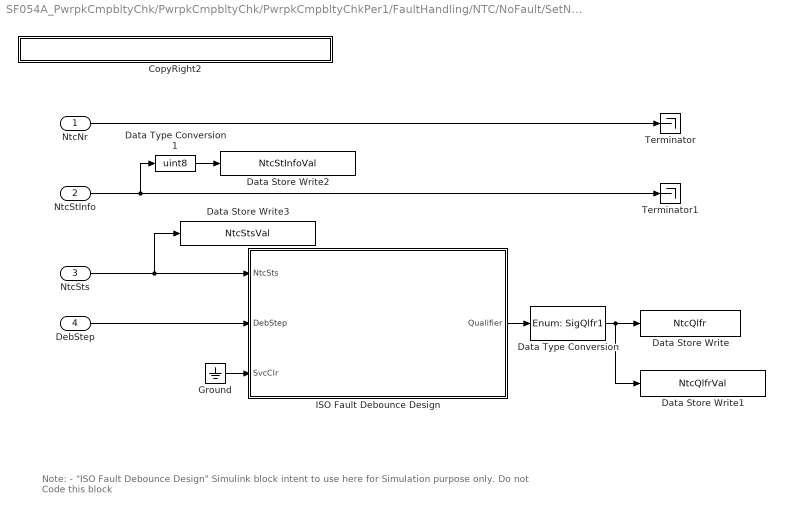
== system SF054A_PwrpkCmpbltyChk/PwrpkCmpbltyChk/PwrpkCmpbltyChkPer1/FaultHandling/NTC/NoFault/SetNtcSts ==
  note: Note:
      |
      | - "ISO Fault Debounce Design" Simulink block intent to use here for Simulation purpose only. Do not Code this block
  NtcNr : Inport
  NtcStInfo : Inport  Port=2
  NtcSts : Inport  Port=3
  DebStep : Inport  Port=4
  CopyRight2 : Subsystem  Description=|  mask(Copyright Information){none=on}
      | Copyright info block.                                               
      |                                                                     
      | Place copyright information at the top of every subsystem in design.
      mask prompts: none "No parameters"
      mask help: Place copyright information at the top of every subsystem in design.
      mask Display:
      | NxtrConf = 'Nexteer Confidential';
      | 
      | sys = bdroot; %handle for the current model ("system")
      | first = get_param(sys,'Created');
      | if(isempty(first))
      |     first = datestr(now,'yyyy');
      | else
      |     first = first(end-3:end);  %year is last four digits
      | end
      | 
      | last = get_param(sys,'LastModifiedDate');
      | if isempty(last)
      |     last = datestr(now,'yyyy');
      | else
      |     last = last(end-3:end);
      | end
      | 
      | if strcmp(first,last)
      |     fprintf('%s -- Copyright %s Nexteer',NxtrConf,first)
      | else
      |     fprintf('%s -- %s%s- %s Nexteer',NxtrConf,char(169),first,last)
      | end
  Data Store Write : DataStoreWrite  DataStoreName=NtcQlfr
  Data Store Write1 : DataStoreWrite  DataStoreName=NtcQlfrVal
  Data Store Write2 : DataStoreWrite  DataStoreName=NtcStInfoVal
  Data Store Write3 : DataStoreWrite  DataStoreName=NtcStsVal
  Data Type Conversion : DataTypeConversion  OutDataTypeStr=Enum: SigQlfr1
  Data Type Conversion1 : DataTypeConversion  OutDataTypeStr=uint8
  Ground : Ground
  ISO Fault Debounce Design : Stateflow chart  TreatAsAtomicUnit=on
      settings: AttributesFormatString=|
      | Simulation Purpose Only.
      | Do Not Code this block
      | Diagnostic Manager Owns this requirement
  Terminator : Terminator
  Terminator1 : Terminator
  wires:
  Data Type Conversion1/1 -> Data Store Write2/1
  NtcStInfo/1 -> Terminator1/1, Data Type Conversion1/1
  NtcSts/1 -> ISO Fault Debounce Design/1(NtcSts), Data Store Write3/1
  Data Type Conversion/1 -> Data Store Write/1, Data Store Write1/1
  Ground/1 -> ISO Fault Debounce Design/3(SvcClr)
  ISO Fault Debounce Design/1(Qualifier) -> Data Type Conversion/1
  DebStep/1 -> ISO Fault Debounce Design/2(DebStep)
  NtcNr/1 -> Terminator/1
